simulink model "uniaxial_table_TransFunc"  (R2023b)
settings: Solver=ode45  StartTime=0.0  StopTime=ddx(end,1)  FixedStep=t_step  MaxStep=t_step  RelTol=1e-6
libraries: cstblocks x1
settings Model: SnapshotInterval=4  Creator=afons  LastModifiedBy=afons

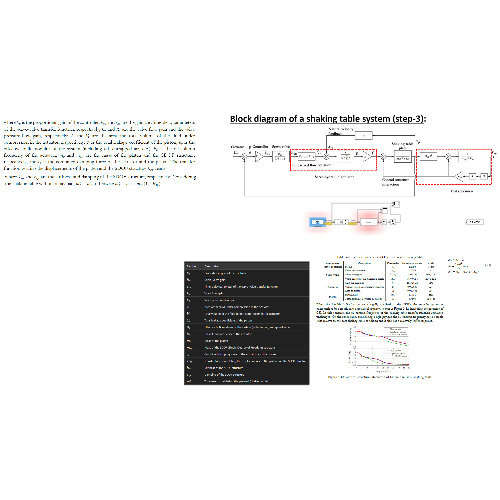
[thumbnail: Simulink's stored preview of the top-level diagram]
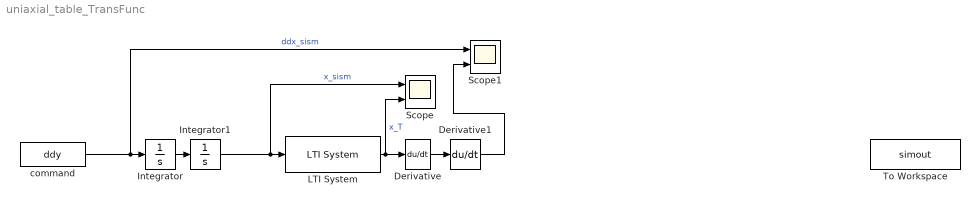
== system uniaxial_table_TransFunc ==
  Derivative : Derivative
  Derivative1 : Derivative
  Integrator : Integrator
  Integrator1 : Integrator
  LTI System : cstblocks/LTI System  sys=Gxraf  IC=[]  PadeOrder=0
  Scope : Scope  NumInputPorts=2
  Scope1 : Scope  NumInputPorts=2
  To Workspace : ToWorkspace  VariableName=simout  SaveFormat=Timeseries  SampleTime=-1
  command : FromWorkspace  VariableName=ddy
  wires:
  command/1 -> Scope1/1, Integrator/1  "ddx_sism"
  Integrator/1 -> Integrator1/1
  Integrator1/1 -> LTI System/1, Scope/1  "x_sism"
  LTI System/1 -> Scope/2, Derivative/1  "x_T"
  Derivative/1 -> Derivative1/1
  Derivative1/1 -> Scope1/2
